simulink model "gnc"  (R2023a)
settings: Solver=ode4  StartTime=0.0  StopTime=10.0  FixedStep=dt_gnc  RelTol=1e-3
settings Model: Creator=ndelurgio  LastModifiedBy=ndelurgio
settings DebuggingCC: ModelReferenceExtraNoncontSigs=warning

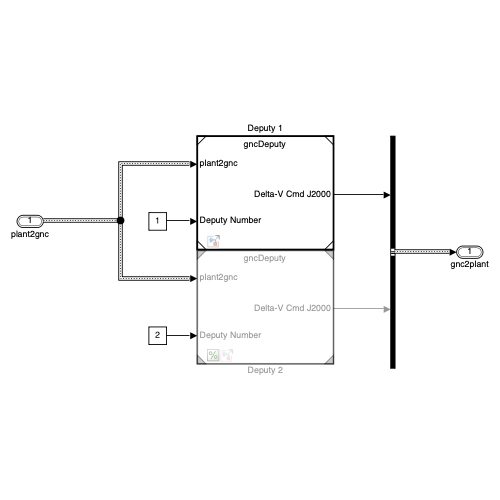
[thumbnail: Simulink's stored preview of the top-level diagram]
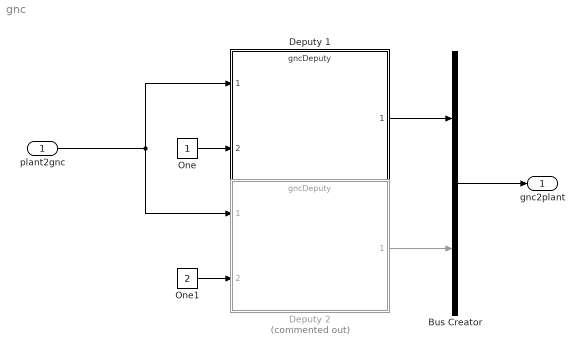
== system gnc ==
  plant2gnc : Inport  OutDataTypeStr=Bus: plant2gnc  BusOutputAsStruct=on
  Bus Creator : BusCreator  Inputs=2  OutDataTypeStr=Bus: gnc2plant  NonVirtualBus=on
      settings: InheritFromInputs=off
  Deputy 1 : ModelReference  ModelNameDialog=gncDeputy  SimulationMode=Normal  ModelReferenceVersion=1.37
  Deputy 2 : ModelReference  Commented=on  ModelNameDialog=gncDeputy  SimulationMode=Normal  ModelReferenceVersion=1.37
  One : Constant  OutDataTypeStr=Inherit: Inherit via back propagation
  One1 : Constant  Value=2  OutDataTypeStr=Inherit: Inherit via back propagation
  gnc2plant : Outport  OutDataTypeStr=Bus: gnc2plant
  wires:
  Deputy 1/1 -> Bus Creator/1
  Deputy 2/1 -> Bus Creator/2
  Bus Creator/1 -> gnc2plant/1
  plant2gnc/1 -> Deputy 2/1, Deputy 1/1
  One/1 -> Deputy 1/2
  One1/1 -> Deputy 2/2
